simulink model "amplifierboard"  (R2020b)
settings: Solver=FixedStepDiscrete  StartTime=0.0  StopTime=2  FixedStep=0.01  RelTol=1e-3
InitFcn:
  | mbd_s32k_consistency_checks(bdroot(gcs));
undefined symbols (not defined in the file): AutoLowerVal, AutoRaiseVal, HoldVal, LED_En, LED_Off, LED_On, Logic_High, Logic_Low, LQFP, ManualLowerVal, ManualRaiseVal, PWRWNDW_CHDLCK, sC_bool_PWMEN, sC_cnt_FWSetting, sC_cnt_Mtr_DrvNo_HB, sC_cnt_PWMHB1to4, sC_cnt_PWMHB5to8, sC_cnt_TargetSlowRange, sC_pct_ManualMax, sC_pct_RampDwn, sC_pct_RampUp, sC_pct_StartPWM, sC_pct_Targetmax, SwitchPackRangeOffset, Threshold_Value, Tolerant_Time
libraries: mbd_s32k1xx_ec_toolbox x205, simulink x59, canmsglib x19, Filter x15, wndwcmd x3
(part 5 of 6)

== system amplifierboard/CAN_Pack_And_Send/RRWndwCntDetect/SwtchPosDetect/RR_Dwn_CntDetect ==
  In6 : Inport
  Data Store Read3 : DataStoreRead  DataStoreName=RR_WindSw_Dwn_Cnts_Low
  Data Store Read4 : DataStoreRead  DataStoreName=RR_WindSw_Dwn_Cnts_Hi
  Logical Operator6 : Logic  AllPortsSameDT=off  OutDataTypeStr=boolean
  Relational Operator11 : RelationalOperator  Operator=<=  OutDataTypeStr=boolean  RndMeth=Simplest
  Relational Operator13 : RelationalOperator  OutDataTypeStr=boolean  RndMeth=Simplest
  Out6 : Outport
  wires:
  Logical Operator6/1 -> Out6/1  "Out"
  Data Store Read4/1 -> Relational Operator11/2
  Data Store Read3/1 -> Relational Operator13/2
  Relational Operator13/1 -> Logical Operator6/2
  Relational Operator11/1 -> Logical Operator6/1
  In6/1 -> Relational Operator11/1, Relational Operator13/1  "In"

== system amplifierboard/CAN_Pack_And_Send/RRWndwCntDetect/SwtchPosDetect/RR_ExpDwn_CntDetect ==
  SwitchCount1 : Inport
  Data Store Read1 : DataStoreRead  DataStoreName=RR_WindSw_ExpDwn_Cnts_Low
  Data Store Read2 : DataStoreRead  DataStoreName=RR_WindSw_ExpDwn_Cnts_Hi
  Logical Operator5 : Logic  AllPortsSameDT=off  OutDataTypeStr=boolean
  Relational Operator10 : RelationalOperator  Operator=<=  OutDataTypeStr=boolean  RndMeth=Simplest
  Relational Operator12 : RelationalOperator  OutDataTypeStr=boolean  RndMeth=Simplest
  Out5 : Outport
  wires:
  Data Store Read1/1 -> Relational Operator12/2
  SwitchCount1/1 -> Relational Operator10/1, Relational Operator12/1  "In"
  Relational Operator10/1 -> Logical Operator5/1
  Data Store Read2/1 -> Relational Operator10/2
  Logical Operator5/1 -> Out5/1  "Out"
  Relational Operator12/1 -> Logical Operator5/2

== system amplifierboard/CAN_Pack_And_Send/RRWndwCntDetect/SwtchPosDetect/RR_ExpUp_CntDetect ==
  In7 : Inport
  Data Store Read5 : DataStoreRead  DataStoreName=RR_WindSw_ExpUp_Cnts_Low
  Data Store Read6 : DataStoreRead  DataStoreName=RR_WindSw_ExpUp_Cnts_Hi
  Logical Operator7 : Logic  AllPortsSameDT=off  OutDataTypeStr=boolean
  Relational Operator14 : RelationalOperator  Operator=<=  OutDataTypeStr=boolean  RndMeth=Simplest
  Relational Operator15 : RelationalOperator  OutDataTypeStr=boolean  RndMeth=Simplest
  AutoRaiseCnt : Outport
  wires:
  Data Store Read5/1 -> Relational Operator15/2
  Relational Operator15/1 -> Logical Operator7/2
  Data Store Read6/1 -> Relational Operator14/2
  In7/1 -> Relational Operator14/1, Relational Operator15/1  "In"
  Logical Operator7/1 -> AutoRaiseCnt/1  "Out"
  Relational Operator14/1 -> Logical Operator7/1

== system amplifierboard/CAN_Pack_And_Send/RRWndwCntDetect/SwtchPosDetect/RR_NrmOpen_CntDetect ==
  In9 : Inport
  Data Store Read10 : DataStoreRead  DataStoreName=RR_WindSw_NrmOpen_Cnts_Hi
  Data Store Read9 : DataStoreRead  DataStoreName=RR_WindSw_NrmOpen_Cnts_Low
  Logical Operator9 : Logic  AllPortsSameDT=off  OutDataTypeStr=boolean
  Relational Operator18 : RelationalOperator  Operator=<=  OutDataTypeStr=boolean  RndMeth=Simplest
  Relational Operator19 : RelationalOperator  OutDataTypeStr=boolean  RndMeth=Simplest
  HoldCnt : Outport
  wires:
  Relational Operator19/1 -> Logical Operator9/2
  Data Store Read9/1 -> Relational Operator19/2
  Relational Operator18/1 -> Logical Operator9/1
  Data Store Read10/1 -> Relational Operator18/2
  Logical Operator9/1 -> HoldCnt/1  "Out"
  In9/1 -> Relational Operator18/1, Relational Operator19/1  "In"

== system amplifierboard/CAN_Pack_And_Send/RRWndwCntDetect/SwtchPosDetect/RR_Up_CntDetect ==
  In8 : Inport
  Data Store Read7 : DataStoreRead  DataStoreName=RR_WindSw_Up_Cnts_Low
  Data Store Read8 : DataStoreRead  DataStoreName=RR_WindSw_Up_Cnts_Hi
  Logical Operator8 : Logic  AllPortsSameDT=off  OutDataTypeStr=boolean
  Relational Operator16 : RelationalOperator  Operator=<=  OutDataTypeStr=boolean  RndMeth=Simplest
  Relational Operator17 : RelationalOperator  OutDataTypeStr=boolean  RndMeth=Simplest
  Out8 : Outport
  wires:
  Relational Operator16/1 -> Logical Operator8/1
  Logical Operator8/1 -> Out8/1  "Out"
  Data Store Read8/1 -> Relational Operator16/2
  Data Store Read7/1 -> Relational Operator17/2
  In8/1 -> Relational Operator16/1, Relational Operator17/1  "In"
  Relational Operator17/1 -> Logical Operator8/2

== system amplifierboard/CAN_Pack_And_Send/RRWndwCntDetect/SwtchPosDetect/SwitchPosDetect1 ==
  ManRaiseCnt : Inport
  ManLowerCnt : Inport  Port=2
  AutoRaiseCnt : Inport  Port=3
  AutoLowerCnt : Inport  Port=4
  HoldCnt : Inport  Port=5
  SwitchCount : Inport  Port=6
  AutoLowerVal : Constant  Value=AutoLowerVal
  AutoRaiseVal : Constant  Value=AutoRaiseVal
  HoldVal : Constant  Value=HoldVal
  ManualLowerVal : Constant  Value=ManualLowerVal
  ManualRaiseVal : Constant  Value=ManualRaiseVal
  Switch{,1..4} (5 alike) : Switch  Criteria=u2 ~= 0
  AvgCount : Outport
  wires:
  SwitchCount/1 -> Switch4/3  "SwitchCount"
  Switch4/1 -> Switch3/3
  HoldCnt/1 -> Switch4/2  "HoldCnt"
  ManLowerCnt/1 -> Switch1/2  "ManLowerCnt"
  AutoLowerCnt/1 -> Switch3/2  "AutoLowerCnt"
  Switch/1 -> AvgCount/1  "AvgCount"
  ManRaiseCnt/1 -> Switch/2  "ManRaiseCnt"
  ManualRaiseVal/1 -> Switch/1
  HoldVal/1 -> Switch4/1
  ManualLowerVal/1 -> Switch1/1
  AutoLowerVal/1 -> Switch3/1
  AutoRaiseVal/1 -> Switch2/1
  Switch3/1 -> Switch2/3
  Switch2/1 -> Switch1/3
  Switch1/1 -> Switch/3
  AutoRaiseCnt/1 -> Switch2/2  "AutoRaiseCnt"

== system amplifierboard/CAN_Receive_And_Unpack/Subsystem/Chart/CalibrateSwitchPack.ReadSwitchAtUpPosition/Generate_Data ==
  Constant1 : Constant  Value=0x00  OutDataTypeStr=uint8
  Constant2 : Constant  Value=0x04  OutDataTypeStr=uint8
  Constant3 : Constant  Value=0x71  OutDataTypeStr=uint8
  Constant4 : Constant  Value=0x01  OutDataTypeStr=uint8
  Constant5 : Constant  Value=0xA1  OutDataTypeStr=uint8
  Constant6 : Constant  Value=0x04  OutDataTypeStr=uint8
  Constant7 : Constant  Value=0x55  OutDataTypeStr=uint8
  Constant8 : Constant  Value=0x55  OutDataTypeStr=uint8
  Mux : Mux  Inputs=8
  Width : Width  DataType=uint8
  Data : Outport
  Length : Outport  Port=2
  wires:
  Mux/1 -> Width/1, Data/1
  Constant2/1 -> Mux/1
  Constant3/1 -> Mux/2
  Constant5/1 -> Mux/4
  Constant1/1 -> Mux/5
  Constant4/1 -> Mux/3
  Constant6/1 -> Mux/6
  Constant7/1 -> Mux/7
  Constant8/1 -> Mux/8
  Width/1 -> Length/1

== system amplifierboard/CAN_Receive_And_Unpack/Subsystem/Chart/CalibrateSwitchPack.SendPos31Response/Generate_Data ==
  Constant1 : Constant  Value=0x02  OutDataTypeStr=uint8
  Constant2 : Constant  Value=0x04  OutDataTypeStr=uint8
  Constant3 : Constant  Value=0x71  OutDataTypeStr=uint8
  Constant4 : Constant  Value=0x01  OutDataTypeStr=uint8
  Constant5 : Constant  Value=0xA1  OutDataTypeStr=uint8
  Constant6 : Constant  Value=0x55  OutDataTypeStr=uint8
  Constant7 : Constant  Value=0x55  OutDataTypeStr=uint8
  Constant8 : Constant  Value=0x55  OutDataTypeStr=uint8
  Mux : Mux  Inputs=8
  Width : Width  DataType=uint8
  Data : Outport
  Length : Outport  Port=2
  wires:
  Mux/1 -> Width/1, Data/1
  Constant2/1 -> Mux/1
  Constant3/1 -> Mux/2
  Constant5/1 -> Mux/4
  Constant1/1 -> Mux/5
  Constant4/1 -> Mux/3
  Constant6/1 -> Mux/6
  Constant7/1 -> Mux/7
  Constant8/1 -> Mux/8
  Width/1 -> Length/1

== system amplifierboard/CAN_Receive_And_Unpack/Subsystem/Chart/CalibrateSwitchPack.SendPos31Response2/Generate_Data ==
  Constant1 : Constant  Value=0x02  OutDataTypeStr=uint8
  Constant2 : Constant  Value=0x04  OutDataTypeStr=uint8
  Constant3 : Constant  Value=0x71  OutDataTypeStr=uint8
  Constant4 : Constant  Value=0x01  OutDataTypeStr=uint8
  Constant5 : Constant  Value=0xA1  OutDataTypeStr=uint8
  Constant6 : Constant  Value=0x55  OutDataTypeStr=uint8
  Constant7 : Constant  Value=0x55  OutDataTypeStr=uint8
  Constant8 : Constant  Value=0x55  OutDataTypeStr=uint8
  Mux : Mux  Inputs=8
  Width : Width  DataType=uint8
  Data : Outport
  Length : Outport  Port=2
  wires:
  Mux/1 -> Width/1, Data/1
  Constant2/1 -> Mux/1
  Constant3/1 -> Mux/2
  Constant5/1 -> Mux/4
  Constant1/1 -> Mux/5
  Constant4/1 -> Mux/3
  Constant6/1 -> Mux/6
  Constant7/1 -> Mux/7
  Constant8/1 -> Mux/8
  Width/1 -> Length/1

== system amplifierboard/CAN_Receive_And_Unpack/Subsystem/Chart/CalibrateSwitchPack.SendPos31StopPosResp/Generate_Data ==
  Constant1 : Constant  Value=0x02  OutDataTypeStr=uint8
  Constant2 : Constant  Value=0x04  OutDataTypeStr=uint8
  Constant3 : Constant  Value=0x71  OutDataTypeStr=uint8
  Constant4 : Constant  Value=0x02  OutDataTypeStr=uint8
  Constant5 : Constant  Value=0xA1  OutDataTypeStr=uint8
  Constant6 : Constant  Value=0x55  OutDataTypeStr=uint8
  Constant7 : Constant  Value=0x55  OutDataTypeStr=uint8
  Constant8 : Constant  Value=0x55  OutDataTypeStr=uint8
  Mux : Mux  Inputs=8
  Width : Width  DataType=uint8
  Data : Outport
  Length : Outport  Port=2
  wires:
  Mux/1 -> Width/1, Data/1
  Constant2/1 -> Mux/1
  Constant3/1 -> Mux/2
  Constant5/1 -> Mux/4
  Constant1/1 -> Mux/5
  Constant4/1 -> Mux/3
  Constant6/1 -> Mux/6
  Constant7/1 -> Mux/7
  Constant8/1 -> Mux/8
  Width/1 -> Length/1

== system amplifierboard/CAN_Receive_And_Unpack/Subsystem/Chart/SendNeg2EResponse/Generate_Data ==
  Constant{1,6..8} (4 alike) : Constant  Value=0x55  OutDataTypeStr=uint8
  Constant2 : Constant  Value=0x03  OutDataTypeStr=uint8
  Constant3 : Constant  Value=0x7F  OutDataTypeStr=uint8
  Constant4 : Constant  Value=0x2E  OutDataTypeStr=uint8
  Constant5 : Constant  Value=0x12  OutDataTypeStr=uint8
  Mux : Mux  Inputs=8
  Width : Width  DataType=uint8
  Data : Outport
  Length : Outport  Port=2
  wires:
  Mux/1 -> Width/1, Data/1
  Constant2/1 -> Mux/1
  Constant3/1 -> Mux/2
  Constant5/1 -> Mux/4
  Constant1/1 -> Mux/5
  Constant4/1 -> Mux/3
  Constant6/1 -> Mux/6
  Constant7/1 -> Mux/7
  Constant8/1 -> Mux/8
  Width/1 -> Length/1

== system amplifierboard/CAN_Receive_And_Unpack/Subsystem/Chart/SendPos11Resp/Generate_Data ==
  Constant{1,5..8} (5 alike) : Constant  Value=0x55  OutDataTypeStr=uint8
  Constant2 : Constant  Value=0x02  OutDataTypeStr=uint8
  Constant3 : Constant  Value=0x51  OutDataTypeStr=uint8
  Constant4 : Constant  Value=0x02  OutDataTypeStr=uint8
  Mux : Mux  Inputs=8
  Width : Width  DataType=uint8
  Data : Outport
  Length : Outport  Port=2
  wires:
  Mux/1 -> Width/1, Data/1
  Constant2/1 -> Mux/1
  Constant3/1 -> Mux/2
  Constant5/1 -> Mux/4
  Constant1/1 -> Mux/5
  Constant4/1 -> Mux/3
  Constant6/1 -> Mux/6
  Constant7/1 -> Mux/7
  Constant8/1 -> Mux/8
  Width/1 -> Length/1

== system amplifierboard/CAN_Receive_And_Unpack/Subsystem/Chart/SendPos22Resp_SW_Ver/Generate_Data ==
  Constant2 : Constant  Value=0x0B  OutDataTypeStr=uint8
  Constant3 : Constant  Value=0x62  OutDataTypeStr=uint8
  Constant4 : Constant  Value=0x01  OutDataTypeStr=uint8
  Constant5 : Constant  Value=0x00  OutDataTypeStr=uint8
  DataMemRead : mbd_s32k1xx_ec_toolbox/Utility Blocks/DataMemRead  base=0x1FFFFFF0  offset=0x0000  ptr=uint8_t
  DataMemRead1 : mbd_s32k1xx_ec_toolbox/Utility Blocks/DataMemRead  base=0x1FFFFFF0  offset=0x0001  ptr=uint8_t
  DataMemRead2 : mbd_s32k1xx_ec_toolbox/Utility Blocks/DataMemRead  base=0x1FFFFFF0  offset=0x0002  ptr=uint8_t
  DataMemRead3 : mbd_s32k1xx_ec_toolbox/Utility Blocks/DataMemRead  base=0x1FFFFFF0  offset=0x0003  ptr=uint8_t
  Mux : Mux  Inputs=8
  Width : Width  DataType=uint8
  Data : Outport
  Length : Outport  Port=2
  wires:
  Mux/1 -> Width/1, Data/1
  Constant2/1 -> Mux/1
  Constant3/1 -> Mux/2
  Constant5/1 -> Mux/4
  DataMemRead/1 -> Mux/5
  Constant4/1 -> Mux/3
  DataMemRead1/1 -> Mux/6
  DataMemRead2/1 -> Mux/7
  DataMemRead3/1 -> Mux/8
  Width/1 -> Length/1

== system amplifierboard/CAN_Receive_And_Unpack/Subsystem/Chart/SendPos22Resp_SW_Ver1/Generate_Data ==
  Constant1 : Constant  Value=0x55  OutDataTypeStr=uint8
  Constant2 : Constant  Value=0x30  OutDataTypeStr=uint8
  Constant3 : Constant  Value=0x55  OutDataTypeStr=uint8
  Constant5 : Constant  Value=0x55  OutDataTypeStr=uint8
  DataMemRead4 : mbd_s32k1xx_ec_toolbox/Utility Blocks/DataMemRead  base=0x1FFFFFF0  offset=0x0004  ptr=uint8_t
  DataMemRead5 : mbd_s32k1xx_ec_toolbox/Utility Blocks/DataMemRead  base=0x1FFFFFF0  offset=0x0005  ptr=uint8_t
  DataMemRead6 : mbd_s32k1xx_ec_toolbox/Utility Blocks/DataMemRead  base=0x1FFFFFF0  offset=0x0006  ptr=uint8_t
  DataMemRead7 : mbd_s32k1xx_ec_toolbox/Utility Blocks/DataMemRead  base=0x1FFFFFF0  offset=0x0007  ptr=uint8_t
  Mux : Mux  Inputs=8
  Width : Width  DataType=uint8
  Data : Outport
  Length : Outport  Port=2
  wires:
  Mux/1 -> Width/1, Data/1
  Constant2/1 -> Mux/1
  Width/1 -> Length/1
  DataMemRead4/1 -> Mux/2
  DataMemRead6/1 -> Mux/4
  DataMemRead7/1 -> Mux/5
  DataMemRead5/1 -> Mux/3
  Constant5/1 -> Mux/8
  Constant3/1 -> Mux/7
  Constant1/1 -> Mux/6

== system amplifierboard/CAN_Receive_And_Unpack/Subsystem/Chart/SendPos2EResponse/Generate_Data ==
  Constant{1,6..8} (4 alike) : Constant  Value=0x55  OutDataTypeStr=uint8
  Constant2 : Constant  Value=0x03  OutDataTypeStr=uint8
  Constant3 : Constant  Value=0x6E  OutDataTypeStr=uint8
  Constant4 : Constant  Value=0x01  OutDataTypeStr=uint8
  Constant5 : Constant  Value=0x01  OutDataTypeStr=uint8
  Mux : Mux  Inputs=8
  Width : Width  DataType=uint8
  Data : Outport
  Length : Outport  Port=2
  wires:
  Mux/1 -> Width/1, Data/1
  Constant2/1 -> Mux/1
  Constant3/1 -> Mux/2
  Constant5/1 -> Mux/4
  Constant1/1 -> Mux/5
  Constant4/1 -> Mux/3
  Constant6/1 -> Mux/6
  Constant7/1 -> Mux/7
  Constant8/1 -> Mux/8
  Width/1 -> Length/1

== system amplifierboard/CAN_Receive_And_Unpack/Subsystem/Chart/SendPos31StopPosResp/Generate_Data ==
  Constant1 : Constant  Value=0x02  OutDataTypeStr=uint8
  Constant2 : Constant  Value=0x04  OutDataTypeStr=uint8
  Constant3 : Constant  Value=0x71  OutDataTypeStr=uint8
  Constant4 : Constant  Value=0x02  OutDataTypeStr=uint8
  Constant5 : Constant  Value=0xA1  OutDataTypeStr=uint8
  Constant6 : Constant  Value=0x55  OutDataTypeStr=uint8
  Constant7 : Constant  Value=0x55  OutDataTypeStr=uint8
  Constant8 : Constant  Value=0x55  OutDataTypeStr=uint8
  Mux : Mux  Inputs=8
  Width : Width  DataType=uint8
  Data : Outport
  Length : Outport  Port=2
  wires:
  Mux/1 -> Width/1, Data/1
  Constant2/1 -> Mux/1
  Constant3/1 -> Mux/2
  Constant5/1 -> Mux/4
  Constant1/1 -> Mux/5
  Constant4/1 -> Mux/3
  Constant6/1 -> Mux/6
  Constant7/1 -> Mux/7
  Constant8/1 -> Mux/8
  Width/1 -> Length/1

== system amplifierboard/CAN_Receive_And_Unpack/Subsystem1/Fold_Unfold/If Action Subsystem ==
  Action Port : ActionPort  ActionPortLabel=if(u1 == 1)
  Forward : Constant  OutDataTypeStr=int8
  "Forward_Direction " : Outport
  wires:
  Forward/1 -> "Forward_Direction "/1

== system amplifierboard/CAN_Receive_And_Unpack/Subsystem1/Fold_Unfold/If Action Subsystem1 ==
  Action Port : ActionPort  ActionPortLabel=elseif(u2 == 1)
  Reverse : Constant  Value=-1  OutDataTypeStr=int8
  Reverse_Direction : Outport
  wires:
  Reverse/1 -> Reverse_Direction/1

== system amplifierboard/CAN_Receive_And_Unpack/Subsystem1/Fold_Unfold/If Action Subsystem2 ==
  Action Port : ActionPort  ActionPortLabel=elseif( u3 == 1 )
  Standstill : Constant  Value=0  OutDataTypeStr=int8
  Standstill_Invalid : Outport
  wires:
  Standstill/1 -> Standstill_Invalid/1

== system amplifierboard/CAN_Receive_And_Unpack/Subsystem1/Fold_Unfold/If Action Subsystem3 ==
  Action Port : ActionPort  ActionPortLabel=elseif( u4 == 1 )
  Standstill : Constant  Value=0  OutDataTypeStr=int8
  Standstill_invalid : Outport
  wires:
  Standstill/1 -> Standstill_invalid/1

== system amplifierboard/CAN_Receive_And_Unpack/Subsystem1/Motor4/If Action Subsystem ==
  Action Port : ActionPort  ActionPortLabel=if(u1 == 1)
  Forward : Constant  OutDataTypeStr=int8
  "Forward_Direction " : Outport
  wires:
  Forward/1 -> "Forward_Direction "/1

== system amplifierboard/CAN_Receive_And_Unpack/Subsystem1/Motor4/If Action Subsystem1 ==
  Action Port : ActionPort  ActionPortLabel=elseif(u2 == 1)
  Reverse : Constant  Value=-1  OutDataTypeStr=int8
  Reverse_Direction : Outport
  wires:
  Reverse/1 -> Reverse_Direction/1

== system amplifierboard/CAN_Receive_And_Unpack/Subsystem1/Motor4/If Action Subsystem2 ==
  Action Port : ActionPort  ActionPortLabel=elseif( u3 == 1 )
  Standstill : Constant  Value=0  OutDataTypeStr=int8
  Standstill_Invalid : Outport
  wires:
  Standstill/1 -> Standstill_Invalid/1

== system amplifierboard/CAN_Receive_And_Unpack/Subsystem1/Motor4/If Action Subsystem3 ==
  Action Port : ActionPort  ActionPortLabel=elseif( u4 == 1 )
  Standstill : Constant  Value=0  OutDataTypeStr=int8
  Standstill_invalid : Outport
  wires:
  Standstill/1 -> Standstill_invalid/1

== system amplifierboard/CAN_Receive_And_Unpack/Subsystem1/Motor5/If Action Subsystem ==
  Action Port : ActionPort  ActionPortLabel=if(u2 == 1)
  Forward : Constant  Value=-1  OutDataTypeStr=int8
  "Forward_Direction " : Outport
  wires:
  Forward/1 -> "Forward_Direction "/1

== system amplifierboard/CAN_Receive_And_Unpack/Subsystem1/Motor5/If Action Subsystem1 ==
  Action Port : ActionPort  ActionPortLabel=else
  Standstill : Constant  Value=0  OutDataTypeStr=int8
  Standstill_Invalid : Outport
  wires:
  Standstill/1 -> Standstill_Invalid/1

== system amplifierboard/CAN_Receive_And_Unpack/Subsystem1/Motor6/If Action Subsystem ==
  Action Port : ActionPort  ActionPortLabel=if(u1 == 1)
  Forward : Constant  OutDataTypeStr=int8
  "Forward_Direction " : Outport
  wires:
  Forward/1 -> "Forward_Direction "/1

== system amplifierboard/CAN_Receive_And_Unpack/Subsystem1/Motor6/If Action Subsystem1 ==
  Action Port : ActionPort  ActionPortLabel=elseif(u2 == 1)
  Reverse : Constant  Value=-1  OutDataTypeStr=int8
  Reverse_Direction : Outport
  wires:
  Reverse/1 -> Reverse_Direction/1

== system amplifierboard/CAN_Receive_And_Unpack/Subsystem1/Motor6/If Action Subsystem2 ==
  Action Port : ActionPort  ActionPortLabel=elseif( u3 == 1 )
  Standstill : Constant  Value=0  OutDataTypeStr=int8
  Standstill_Invalid : Outport
  wires:
  Standstill/1 -> Standstill_Invalid/1

== system amplifierboard/CAN_Receive_And_Unpack/Subsystem1/Motor6/If Action Subsystem3 ==
  Action Port : ActionPort  ActionPortLabel=elseif( u4 == 1 )
  Standstill : Constant  Value=0  OutDataTypeStr=int8
  Standstill_invalid : Outport
  wires:
  Standstill/1 -> Standstill_invalid/1

== system amplifierboard/CAN_Receive_And_Unpack/Subsystem1/Subsystem1/Motor2 ==
  Input : Inport
  Input1 : Inport  Port=2
  Compare To Constant : simulink/Logic and Bit Operations/Compare To Constant  relop===  const=1.0  OutDataTypeStr=boolean
  Compare To Constant{1..2,4..5} (4 alike) : simulink/Logic and Bit Operations/Compare To Constant  relop===  const=0  OutDataTypeStr=boolean
  Compare To Constant3 : simulink/Logic and Bit Operations/Compare To Constant  relop===  const=1  OutDataTypeStr=boolean
  Compare To Constant6 : simulink/Logic and Bit Operations/Compare To Constant  relop===  const=1  OutDataTypeStr=boolean
  Compare To Constant7 : simulink/Logic and Bit Operations/Compare To Constant  relop===  const=1  OutDataTypeStr=boolean
  If : If  NumInputs=4  IfExpression=u1 == 1  ElseIfExpressions=u2 == 1, u3 == 1 , u4 == 1  ShowElse=off
  If Action Subsystem : Subsystem  TreatAsAtomicUnit=on
  If Action Subsystem1 : Subsystem  TreatAsAtomicUnit=on
  If Action Subsystem2 : Subsystem  TreatAsAtomicUnit=on
  If Action Subsystem3 : Subsystem  TreatAsAtomicUnit=on
  Logical Operator{,1..3} (4 alike) : Logic  AllPortsSameDT=off  OutDataTypeStr=boolean
  Merge : Merge  Inputs=4
  Motor : Outport
  wires:
  Logical Operator/1 -> If/1
  If/3 -> If Action Subsystem2/Action
  Compare To Constant1/1 -> Logical Operator/2
  Logical Operator1/1 -> If/2
  Logical Operator2/1 -> If/3
  If/1 -> If Action Subsystem/Action
  If Action Subsystem2/1(Standstill_Invalid) -> Merge/3
  If Action Subsystem3/1(Standstill_invalid) -> Merge/4
  If Action Subsystem1/1(Reverse_Direction) -> Merge/2
  Merge/1 -> Motor/1
  Compare To Constant6/1 -> Logical Operator3/1
  If/4 -> If Action Subsystem3/Action
  Compare To Constant7/1 -> Logical Operator3/2
  Input/1 -> Compare To Constant/1, Compare To Constant6/1, Compare To Constant4/1, Compare To Constant2/1
  Logical Operator3/1 -> If/4
  Compare To Constant/1 -> Logical Operator/1
  Compare To Constant3/1 -> Logical Operator1/2
  Compare To Constant4/1 -> Logical Operator2/1
  Compare To Constant2/1 -> Logical Operator1/1
  If/2 -> If Action Subsystem1/Action
  If Action Subsystem/1("Forward_Direction ") -> Merge/1
  Compare To Constant5/1 -> Logical Operator2/2
  Input1/1 -> Compare To Constant1/1, Compare To Constant3/1, Compare To Constant5/1, Compare To Constant7/1

== system amplifierboard/CAN_Receive_And_Unpack/Subsystem1/Subsystem1/Motor3 ==
  Input : Inport
  Input1 : Inport  Port=2
  Compare To Constant : simulink/Logic and Bit Operations/Compare To Constant  relop===  const=1.0  OutDataTypeStr=boolean
  Compare To Constant{1..2,4..5} (4 alike) : simulink/Logic and Bit Operations/Compare To Constant  relop===  const=0  OutDataTypeStr=boolean
  Compare To Constant3 : simulink/Logic and Bit Operations/Compare To Constant  relop===  const=1  OutDataTypeStr=boolean
  Compare To Constant6 : simulink/Logic and Bit Operations/Compare To Constant  relop===  const=1  OutDataTypeStr=boolean
  Compare To Constant7 : simulink/Logic and Bit Operations/Compare To Constant  relop===  const=1  OutDataTypeStr=boolean
  If : If  NumInputs=4  IfExpression=u1 == 1  ElseIfExpressions=u2 == 1, u3 == 1 , u4 == 1  ShowElse=off
  If Action Subsystem : Subsystem  TreatAsAtomicUnit=on
  If Action Subsystem1 : Subsystem  TreatAsAtomicUnit=on
  If Action Subsystem2 : Subsystem  TreatAsAtomicUnit=on
  If Action Subsystem3 : Subsystem  TreatAsAtomicUnit=on
  Logical Operator{,1..3} (4 alike) : Logic  AllPortsSameDT=off  OutDataTypeStr=boolean
  Merge : Merge  Inputs=4
  Motor : Outport
  wires:
  Input1/1 -> Compare To Constant7/1, Compare To Constant5/1, Compare To Constant3/1, Compare To Constant1/1
  Compare To Constant5/1 -> Logical Operator2/2
  If Action Subsystem/1("Forward_Direction ") -> Merge/1
  If/2 -> If Action Subsystem1/Action
  Compare To Constant2/1 -> Logical Operator1/1
  Compare To Constant4/1 -> Logical Operator2/1
  Compare To Constant3/1 -> Logical Operator1/2
  Compare To Constant/1 -> Logical Operator/1
  Logical Operator3/1 -> If/4
  Input/1 -> Compare To Constant2/1, Compare To Constant4/1, Compare To Constant6/1, Compare To Constant/1
  Compare To Constant7/1 -> Logical Operator3/2
  If/4 -> If Action Subsystem3/Action
  Compare To Constant6/1 -> Logical Operator3/1
  Merge/1 -> Motor/1
  If Action Subsystem1/1(Reverse_Direction) -> Merge/2
  If Action Subsystem3/1(Standstill_invalid) -> Merge/4
  If Action Subsystem2/1(Standstill_Invalid) -> Merge/3
  If/1 -> If Action Subsystem/Action
  Logical Operator2/1 -> If/3
  Logical Operator1/1 -> If/2
  Compare To Constant1/1 -> Logical Operator/2
  If/3 -> If Action Subsystem2/Action
  Logical Operator/1 -> If/1

== system amplifierboard/Motor_Control/Motor_Control/Chart/SendSPI/Switch Case Action Subsystem ==
  SPI_Command1 : Inport  OutDataTypeStr=uint8  PortDimensions=[1 2]
  Action Port : ActionPort  ActionPortLabel=case [ 1 ]:
  LPSPI_Master_Transfer : mbd_s32k1xx_ec_toolbox/Communication Blocks/SPI Blocks/LPSPI_Master_Transfer  instance=2  pcs=0  pcs_polarity=ActiveLow  xfermode=Blocking  timeout=50  spi_upd=on
  Status_Out1 : Outport  OutDataTypeStr=uint8
  wires:
  SPI_Command1/1 -> LPSPI_Master_Transfer/1
  LPSPI_Master_Transfer/1 -> Status_Out1/1

== system amplifierboard/Motor_Control/Motor_Control/Chart/SendSPI/Switch Case Action Subsystem1 ==
  SPI_Command2 : Inport  OutDataTypeStr=uint8  PortDimensions=[1 2]
  Action Port : ActionPort  ActionPortLabel=case [ 2 ]:
  LPSPI_Master_Transfer : mbd_s32k1xx_ec_toolbox/Communication Blocks/SPI Blocks/LPSPI_Master_Transfer  instance=1  pcs=1  pcs_polarity=ActiveLow  xfermode=Blocking  timeout=50  spi_upd=on
  Status_Out2 : Outport  OutDataTypeStr=uint8
  wires:
  LPSPI_Master_Transfer/1 -> Status_Out2/1
  SPI_Command2/1 -> LPSPI_Master_Transfer/1

== system amplifierboard/CAN_Receive_And_Unpack/Subsystem1/Subsystem1/Motor2/If Action Subsystem ==
  Action Port : ActionPort  ActionPortLabel=if(u1 == 1)
  Forward : Constant  OutDataTypeStr=int8
  "Forward_Direction " : Outport
  wires:
  Forward/1 -> "Forward_Direction "/1

== system amplifierboard/CAN_Receive_And_Unpack/Subsystem1/Subsystem1/Motor2/If Action Subsystem1 ==
  Action Port : ActionPort  ActionPortLabel=elseif(u2 == 1)
  Reverse : Constant  Value=-1  OutDataTypeStr=int8
  Reverse_Direction : Outport
  wires:
  Reverse/1 -> Reverse_Direction/1

== system amplifierboard/CAN_Receive_And_Unpack/Subsystem1/Subsystem1/Motor2/If Action Subsystem2 ==
  Action Port : ActionPort  ActionPortLabel=elseif( u3 == 1 )
  Standstill : Constant  Value=0  OutDataTypeStr=int8
  Standstill_Invalid : Outport
  wires:
  Standstill/1 -> Standstill_Invalid/1

== system amplifierboard/CAN_Receive_And_Unpack/Subsystem1/Subsystem1/Motor2/If Action Subsystem3 ==
  Action Port : ActionPort  ActionPortLabel=elseif( u4 == 1 )
  Standstill : Constant  Value=0  OutDataTypeStr=int8
  Standstill_invalid : Outport
  wires:
  Standstill/1 -> Standstill_invalid/1

== system amplifierboard/CAN_Receive_And_Unpack/Subsystem1/Subsystem1/Motor3/If Action Subsystem ==
  Action Port : ActionPort  ActionPortLabel=if(u1 == 1)
  Forward : Constant  OutDataTypeStr=int8
  "Forward_Direction " : Outport
  wires:
  Forward/1 -> "Forward_Direction "/1

== system amplifierboard/CAN_Receive_And_Unpack/Subsystem1/Subsystem1/Motor3/If Action Subsystem1 ==
  Action Port : ActionPort  ActionPortLabel=elseif(u2 == 1)
  Reverse : Constant  Value=-1  OutDataTypeStr=int8
  Reverse_Direction : Outport
  wires:
  Reverse/1 -> Reverse_Direction/1

== system amplifierboard/CAN_Receive_And_Unpack/Subsystem1/Subsystem1/Motor3/If Action Subsystem2 ==
  Action Port : ActionPort  ActionPortLabel=elseif( u3 == 1 )
  Standstill : Constant  Value=0  OutDataTypeStr=int8
  Standstill_Invalid : Outport
  wires:
  Standstill/1 -> Standstill_Invalid/1

== system amplifierboard/CAN_Receive_And_Unpack/Subsystem1/Subsystem1/Motor3/If Action Subsystem3 ==
  Action Port : ActionPort  ActionPortLabel=elseif( u4 == 1 )
  Standstill : Constant  Value=0  OutDataTypeStr=int8
  Standstill_invalid : Outport
  wires:
  Standstill/1 -> Standstill_invalid/1

== stateflow chart amplifierboard/CAN_Pack_And_Send/Trigger ==
  (default) -> (junction 125)
  (junction 125) -> (junction 127) [order 1] : [TX_Cnt < 5]
      | {TX_Cnt = TX_Cnt + 1;
      | bool_TX = false;}
      | %stop transmit
  (junction 127) -> (junction 92)
  (junction 125) -> (junction 92) [order 2] : {%set up to transmit message
      | bool_TX = true;
      | TX_Cnt = 0;}
  data: TX_Cnt local =0; bool_TX output

== stateflow chart amplifierboard/HALL_Input_Capture/Hall_Count_Calculation ==
  settings: executeAtInitialization=1
  (default) -> (junction 1100) : {Motor_idx = 0;}
  (junction 1100) -> (junction 1104) [order 1] : HE1
      | {Motor_idx = 1;}
  (junction 1100) -> (junction 1102) [order 2]
  (junction 1104) -> (junction 1106)
  (junction 1102) -> (junction 1106) [order 1] : HE2
      | {Motor_idx = 2;}
  (junction 1102) -> (junction 1112) [order 2]
  (junction 1106) -> (junction 1117)
  (junction 1112) -> (junction 1117) [order 1] : HE3
      | {Motor_idx = 3;}
  (junction 1112) -> (junction 1115) [order 2]
  (junction 1117) -> (junction 1111)
  (junction 1115) -> (junction 1111) [order 1] : HE4
      | {Motor_idx = 4;}
  (junction 1115) -> (junction 1126) [order 2]
  (junction 1111) -> (junction 1124)
  (junction 1126) -> (junction 1124) [order 1] : HE5
      | {Motor_idx = 5;}
  (junction 1126) -> (junction 1121) [order 2]
  (junction 1124) -> (junction 1123)
  (junction 1121) -> (junction 1123) [order 1] : HE6
      | {Motor_idx = 6;}
  (junction 1121) -> (junction 1157) [order 2]
  (junction 1123) -> (junction 1155)
  (junction 1157) -> (junction 1155) [order 1] : HE7
      | {Motor_idx = 7;}
  (junction 1157) -> (junction 1158) [order 2]
  (junction 1155) -> (junction 1156)
  (junction 1158) -> (junction 1156) [order 1] : HE8
      | {Motor_idx = 8;}
  (junction 1158) -> (junction 1147) [order 2] : Tick
  (junction 1156) -> (junction 1138) [order 2]
  (junction 1156) -> (junction 1138) [order 1] : [MotorPosCount(Motor_idx) > 1000]
      | {MotorPosRawCount(Motor_idx) = min(MotorPosRawCount(Motor_idx)+1,MotorPosMaxCount(Motor_idx));}
  (junction 1138) -> (junction 1147) [order 1] : [MotorPosCount(Motor_idx) < 0]
      | {MotorPosRawCount(Motor_idx) = max(MotorPosRawCount(Motor_idx)-1, 0);}
  (junction 1138) -> (junction 1147) [order 2]
  (junction 1147) -> (junction 1152) : {MotorPosCount= uint8((single(MotorPosRawCount)./single(MotorPosMaxCount))*254);}
  data: MotorPosCount output uint8 size=8 =zeros(8,1,'uint8'); Motor_idx local size=1 =0; MotorPosRawCount local uint16 size=8 =uint16([100;100;100;100;100;100;100;100]); MotorPosMaxCount local uint16 size=8 =uint16([1000;1000;1000;1000;1000;1000;1000;1000])
  events: HE1 input FUNCTION_CALL_EVENT; HE2 input FUNCTION_CALL_EVENT; HE3 input FUNCTION_CALL_EVENT; HE4 input FUNCTION_CALL_EVENT; HE5 input FUNCTION_CALL_EVENT; HE6 input FUNCTION_CALL_EVENT; HE7 input FUNCTION_CALL_EVENT; Tick input FUNCTION_CALL_EVENT; Trig_HallTrack input FUNCTION_CALL_EVENT; HE8 input FUNCTION_CALL_EVENT

== stateflow chart amplifierboard/Motor_Control/Subsystem/Chart ==
  state Idle
    PWM_Out = zeros(6,1,'single');
  state Assign
    en: PWM_Out = zeros(6,1,'single');
    Assign -> (junction 9) [order 1] : {for_idx = 1;}
    (junction 9) -> (junction 11) [order 1] : [for_idx < 7]
    (junction 11) -> (junction 18) [order 2]
    (junction 18) -> (junction 25) [order 2]
    (junction 25) -> (junction 30) [order 2]
    (junction 15) -> (junction 9) : {for_idx = for_idx + 1;}
    (junction 11) -> (junction 15) [order 1] : [aV_int_MotorDir(for_idx) == 0]
        | { PWM_Out(for_idx) = 0;}
    (junction 18) -> (junction 20) [order 1] : [aV_int_MotorDir(for_idx) == 1]
        | {PWM_Out(for_idx) = min(max((PWM_Out(for_idx)+RampUp),StartPWM),ManualMaxPWM);}
    (junction 25) -> (junction 27) [order 1] : [PositionError(for_idx) < TargetSlowRange]
        | {PWM_Out(for_idx) = max((PWM_Out(for_idx)-RampDwn), StartPWM);}
    (junction 30) -> (junction 32) : {PWM_Out(for_idx) = min(max((PWM_Out(for_idx)+RampUp),StartPWM),TargetMaxPWM);}
    (junction 9) -> (junction 13) [order 2]
    (junction 20) -> (junction 15)
    (junction 27) -> (junction 20)
    (junction 32) -> (junction 27)
  (default) -> Idle
  Idle -> Assign : [any(aV_int_MotorDir ~= 0)]
  Assign -> Idle [order 1] : [all(aV_int_MotorDir == 0)...
      | && all(PWM_Out == 0)]
  data: aV_int_MotorDir input int8 size=6; PositionError input uint8 size=6; PWM_Out output single size=6 =zeros(6,1,'single'); for_idx local size=1 =0; RampUp input single size=1; RampDwn input single size=1; StartPWM input single size=1; ManualMaxPWM input single size=1; TargetMaxPWM input single size=1; TargetSlowRange input uint16 size=1

== stateflow chart amplifierboard/CAN_Receive_And_Unpack/Subsystem/Chart ==
  settings: sampleTime=1
  state Idle
    StateFlowState=0;
  note: ?
  state ParseMessage
    StateFlowState=1;
    ContinueStateProcessing = 1;
  state Diagnostic_ID_req_Verified
    StateFlowState=1;
  state CalibrateSwitchPack
    state AcknowledgeSer31Request
      ContinueStateProcessing = 1;
      StateFlowState= 11;
    state WaitforCommand
      StateFlowState=12;
    state SendPos31Response1
    state SampleNO_SwitchState
      ReadSwitchAtNormOpen
      StateFlowState=13;
    state SendPos31Response [function]
    state CapturingDownSwitchValues
      ReadSwitchAtDownPostion
      StateFlowState=14;
    state ReadSwitchAtNormOpen [function]
    state ReadSwitchAtDownPostion [function]
    state CapturingExpDownSwitchValues
      ReadSwitchAtExpDownPosition
      StateFlowState=15;
    state ReadSwitchAtExpDownPosition [function]
    state CapturingUpSwitchValues
      ReadSwitchAtUpPosition
      StateFlowState=16;
    state ReadSwitchAtUpPosition [function]
    state ReadSwitchAtExpUpPosition [function]
    state SampleExpUp_SwitchState
      ReadSwitchAtExpUpPosition
      StateFlowState=17;
    state SendPos31StopPosResp [function]
    state ExitSer31CalSwPack
      WriteCalValuesToEEPROM
      StateFlowState=18;
    state SendPos31Response2 [function]
    state WriteCalValuesToEEPROM [function]
    state Exit
      StateFlowState=19;
      ContinueStateProcessing = 0;
    (default) -> AcknowledgeSer31Request
    AcknowledgeSer31Request -> WaitforCommand : after(10, msec){SendPos31Response}
    WaitforCommand -> SendPos31Response1 : [ (ServiceID == 0x31) && (ServiceByte0==0x01) && (ServiceByte1==0xA1) && (ServiceByte2==0x02)&& (ServiceByte3 ==0x01) ]{SendPos31Response}
    SendPos31Response1 -> SampleNO_SwitchState : after(10, msec)
    SampleNO_SwitchState -> CapturingDownSwitchValues [order 1] : [ (ServiceID == 0x31) && (ServiceByte0==0x01) && (ServiceByte1==0xA1) && (ServiceByte2==0x02)&& (ServiceByte3 ==0x02) ]{SendPos31Response}
    SampleNO_SwitchState -> ExitSer31CalSwPack [order 2] : [ (ServiceID == 0x31) && (ServiceByte0==0x02) && (ServiceByte1==0xA1) && (ServiceByte2==0x02) ]{SendPos31StopPosResp}
    CapturingDownSwitchValues -> ExitSer31CalSwPack [order 2] : [ (ServiceID == 0x31) && (ServiceByte0==0x02) && (ServiceByte1==0xA1) && (ServiceByte2==0x02) ]{SendPos31StopPosResp}
    CapturingDownSwitchValues -> CapturingExpDownSwitchValues [order 1] : [ (ServiceID == 0x31) && (ServiceByte0==0x01) && (ServiceByte1==0xA1) && (ServiceByte2==0x02)&& (ServiceByte3 ==0x03) ]{SendPos31Response}
    CapturingExpDownSwitchValues -> ExitSer31CalSwPack [order 2] : [ (ServiceID == 0x31) && (ServiceByte0==0x02) && (ServiceByte1==0xA1) && (ServiceByte2==0x02) ]{SendPos31StopPosResp}
    CapturingExpDownSwitchValues -> CapturingUpSwitchValues [order 1] : [ (ServiceID == 0x31) && (ServiceByte0==0x01) && (ServiceByte1==0xA1) && (ServiceByte2==0x02)&& (ServiceByte3 ==0x04) ]{SendPos31Response}
    CapturingUpSwitchValues -> ExitSer31CalSwPack [order 2] : [ (ServiceID == 0x31) && (ServiceByte0==0x02) && (ServiceByte1==0xA1) && (ServiceByte2==0x02) ]{SendPos31StopPosResp}
    CapturingUpSwitchValues -> SampleExpUp_SwitchState [order 1] : [ (ServiceID == 0x31) && (ServiceByte0==0x01) && (ServiceByte1==0xA1) && (ServiceByte2==0x02)&& (ServiceByte3 ==0x05) ]{SendPos31Response2}
    SampleExpUp_SwitchState -> ExitSer31CalSwPack : [ (ServiceID == 0x31) && (ServiceByte0==0x02) && (ServiceByte1==0xA1) && (ServiceByte2==0x02) ]{SendPos31StopPosResp}
    ExitSer31CalSwPack -> Exit : [ (ServiceID == 0x31) && (ServiceByte0==0x03) && (ServiceByte1==0xA1) && (ServiceByte2==0x02) ]
    Exit -> (junction 190)
  state SendNeg2EResponse [function]
  state SW_VersionRequest
    ContinueStateProcessing = 1;
    StateFlowState=9;
  state PositiveRespone
    StateFlowState=2;
  state SendPos2EResponse [function]
  state NegResponse_ID
    StateFlowState=7;
  state VersionSendComplete
    ContinueStateProcessing = 0;
    StateFlowState=10;
  note: ?
  state WaitForSWVersionRequest
    StateFlowState=3;
  state SendPos22Resp_SW_Ver [function]
  state SendPos22Resp_SW_Ver1 [function]
  state SendingSoftwareVersionFirstMsg
    StateFlowState=4;
  state SendingSoftwareVersion2ndMsg
  state SendPos11Resp [function]
  state ExitCal
    ContinueStateProcessing = 0;
    StateFlowState=20;
  state WaitForResetRequest
    StateFlowState=5;
  state ECU_Reset [function]
  state ExitLIN_Testing
    ContinueStateProcessing = 0;
    StateFlowState=32;
  state SendingPosResp_ForResetReq
    StateFlowState=6;
  state SendPos31StopPosResp [function]
  state PerformingECU_Reset
    ECU_Reset
    StateFlowState=7;
  state InitializeLIN_Cntrler
    state WriteMODE  % set to Normal Run mode
      StateFlowState= 29;
      en: LIN_Status = SendSPI_3Byte([uint8(0x10),uint8(0b00000000), uint8(0x80)] );
      en: LIN_Status = SendSPI_3Byte([uint8(0xFF),uint8(0b10000000), uint8(0x00)] );
      en: LIN_Status = SendSPI_3Byte([uint8(0x10),uint8(0b10000000), uint8(0x00)] );
    state WriteLIN1_LCFG1 % set to initialization state, write MBL= 20Bits
      StateFlowState= 29;
      en: LIN_Status = SendSPI_3Byte([uint8(0x30),uint8(0b00000000), uint8(0x01)] );
      en: LIN_Status = SendSPI_3Byte([uint8(0x30),uint8(0b00000000), uint8(0b01111001)] );
      en: LIN_Status = SendSPI_3Byte([uint8(0x30),uint8(0b10000000), uint8(0x00)] )
      %WriteBaudRate set baud rate to 20k
      en: LIN_Status5Byte = SendSPI_5Byte([uint8(0x35),uint8(0b00000010), uint8(0x3), uint8(0x72), uint8(0x00) ] );
      en: LIN_Status5Byte = SendSPI_5Byte([uint8(0x35),uint8(0b10000010), uint8(0x0), uint8(0x0), uint8(0x00) ] );
      ;
    state LIN_Status10Byte = SendSPI(SPI_Command1) [function]
    state LIN_Status = SendSPI_3Byte(SPI_Command1) [function]
    state WritePLLCFG % init for 1.832 Mhz Oscillator in Normal mode
      en: LIN_Status = SendSPI_3Byte([uint8(0x30),uint8(0b00000000), uint8(0x00)] );
      en: LIN_Status = SendSPI_3Byte( [uint8(0x01),uint8(0b00000000), uint8(0x4)] )
      en: LIN_Status = SendSPI_3Byte( [uint8(0x01),uint8(0b10000000), uint8(0x0)] );
    state LIN_Status5Byte = SendSPI_5Byte(SPI_Command1) [function]
    state WriteLIN1_LRTC % set RTO to 14 - it is its default value so this step is not necessary
      en: LIN_Status = SendSPI_3Byte([uint8(0x34),uint8(0b00000000), uint8(0xE)]) ;
      en: LIN_Status = SendSPI_3Byte([uint8(0x34),uint8(0b10000000), uint8(0x0)]) ;
    state WriteLIN1_ID
      en: LIN_Status = SendSPI_3Byte([uint8(0x3A),uint8(0b00000000), uint8(0b00101010)] );
      en: LIN_Status = SendSPI_3Byte([uint8(0x3A),uint8(0b10000000), uint8(0x0)] );
    state WriteLIN1_BUF_CTRL % Data Direction = Master TX, 8 Byte TX, Classic Chksum
      en: LIN_Status = SendSPI_3Byte( [uint8(0x3B),uint8(0b00000000), uint8(0b00011111)] );
      en: LIN_Status = SendSPI_3Byte( [uint8(0x3B),uint8(0b10000000), uint8(0x0)] );
    state WriteLIN1_LBD1
      en: LIN_Status10Byte = SendSPI([uint8(0x53),uint8(0b00000111), uint8(0xAA),uint8(0xAA),...
      uint8(0xAA), uint8(0xAA), uint8(0xAA), uint8(0xAA), uint8(0xAA), uint8(0xAA)]) ;
      en: LIN_Status10Byte = SendSPI([uint8(0x53),uint8(0b10000111), uint8(0x0),uint8(0x0),...
      uint8(0x0), uint8(0x0), uint8(0x0), uint8(0x0), uint8(0x0), uint8(0x0)]) ;
    state WriteLIN1_LCFG2 % set to Normal Mode
      %en: LIN_Status = SendSPI_3Byte([uint8(0x30),uint8(0b00000000), uint8(0x00)] );
      %en: LIN_Status = SendSPI_3Byte([uint8(0x30),uint8(0b10000000), uint8(0x00)] );
      en: LIN_Status = SendSPI_3Byte([uint8(0x11),uint8(0b10000000), uint8(0x00)] );
    state WriteLCOM2_ADDR
      en: LIN_Status = SendSPI_3Byte([uint8(0x21),uint8(0b00000000), uint8(0b00000001)] );
    state WriteLIN1_CNTRL
      en: LIN_Status = SendSPI_3Byte( [uint8(0x39),uint8(0b00000000), uint8(0x01)] );
      en: LIN_Status = SendSPI_3Byte( [uint8(0x39),uint8(0b10000000), uint8(0x00)] );
      %en: LIN_Status = SendSPI_3Byte( [uint8(0x21),uint8(0b00000000), uint8(0x01)] );
      %en: LIN_Status = SendSPI_3Byte( [uint8(0x21),uint8(0b10000000), uint8(0x00)] );
      StateFlowState= 31;
    (default) -> WriteMODE  % set to Normal Run mode
    WriteMODE  % set to Normal Run mode -> WriteLIN1_LCFG1 % set to initialization state, write MBL= 20Bits : after(5, msec)
    WriteLIN1_LCFG1 % set to initialization state, write MBL= 20Bits -> WritePLLCFG % init for 1.832 Mhz Oscillator in Normal mode : after(5, msec)
    WritePLLCFG % init for 1.832 Mhz Oscillator in Normal mode -> WriteLIN1_LRTC % set RTO to 14 - it is its default value so this step is not necessary : after(5, msec)
    WriteLIN1_LRTC % set RTO to 14 - it is its default value so this step is not necessary -> WriteLIN1_ID : after(5, msec)
    WriteLIN1_ID -> WriteLIN1_BUF_CTRL % Data Direction = Master TX, 8 Byte TX, Classic Chksum : after(5, msec)
    WriteLIN1_BUF_CTRL % Data Direction = Master TX, 8 Byte TX, Classic Chksum -> WriteLIN1_LBD1 : after(5, msec)
    WriteLIN1_LBD1 -> WriteLIN1_LCFG2 % set to Normal Mode : after(5, msec)
    WriteLIN1_LCFG2 % set to Normal Mode -> WriteLCOM2_ADDR : after(5, msec)
    WriteLCOM2_ADDR -> WriteLIN1_CNTRL : after(5, msec)
    WriteLIN1_CNTRL -> (junction 301)
  state InitializeLIN_Cntrler1
    state ReadRegister
      en: LIN_Status = SendSPI_3Byte([uint8(ServiceByte2),uint8(0b10000000), uint8(0x00)] );
      StateFlowState= 31;
    state LIN_Status = SendSPI_3Byte(SPI_Command1) [function]
    (default) -> ReadRegister
    ReadRegister -> (junction 362)
  PerformingECU_Reset -> Idle : after(1,sec)
  (default) -> Idle
  VersionSendComplete -> Idle
  NegResponse_ID -> Idle : after(500, msec)
  WaitForSWVersionRequest -> Idle [order 2] : after(5, sec)
  ExitLIN_Testing -> Idle
  ExitCal -> Idle : after(20, msec)
  Idle -> ParseMessage : [NewMsgRXed==1]
  ParseMessage -> CalibrateSwitchPack [order 5] : [ (ServiceID == 0x31) && (ServiceByte0==0x01) && (ServiceByte1==0xA1)&& (ServiceByte2==0x02) ]
  ParseMessage -> Diagnostic_ID_req_Verified [order 1] : [ (ServiceID == 0x2E) && (ServiceByte0==0x01) && (ServiceByte1==0x01) ]
  ParseMessage -> InitializeLIN_Cntrler [order 3] : [ (ServiceID == 0x22) && (ServiceByte0==0x01) && (ServiceByte1==0x01) ]
  ParseMessage -> InitializeLIN_Cntrler1 [order 2] : [ (ServiceID == 0x22) && (ServiceByte0==0x01) && (ServiceByte1==0x02)   ]
  ParseMessage -> SW_VersionRequest [order 4] : [ (ServiceID == 0x22) && (ServiceByte0==0x01) && (ServiceByte1==0x00) ]{SendPos22Resp_SW_Ver}
  Diagnostic_ID_req_Verified -> NegResponse_ID [order 2] : [ (ServiceByte2~=0x17) ]{SendNeg2EResponse}
  Diagnostic_ID_req_Verified -> PositiveRespone [order 1] : [ServiceByte2==0x17]{SendPos2EResponse}
  SW_VersionRequest -> VersionSendComplete : {SendPos22Resp_SW_Ver1}
  CalibrateSwitchPack -> ExitCal : [ (ServiceID == 0x31) && (ServiceByte0==0x03) && (ServiceByte1==0xA1) && (ServiceByte2==0x02) ]{SendPos31StopPosResp}
  PositiveRespone -> WaitForSWVersionRequest : after(20, msec)
  WaitForSWVersionRequest -> SendingSoftwareVersionFirstMsg [order 1] : [ (ServiceID == 0x22) && (ServiceByte0==0x01) && (ServiceByte1==0x00) ]{SendPos22Resp_SW_Ver}
  SendingSoftwareVersionFirstMsg -> SendingSoftwareVersion2ndMsg : {SendPos22Resp_SW_Ver1}
  SendingSoftwareVersion2ndMsg -> WaitForResetRequest : after(20, msec)
  WaitForResetRequest -> SendingPosResp_ForResetReq : [ (ServiceID == 0x11) && (ServiceByte0==0x2)]{SendPos11Resp}
  InitializeLIN_Cntrler1 -> ExitLIN_Testing : [StateFlowState==31]
  InitializeLIN_Cntrler -> ExitLIN_Testing : [StateFlowState==31]
  SendingPosResp_ForResetReq -> PerformingECU_Reset : after(500, msec)
  data: SPI_Command1 function_input uint8 size=[1 10]; LIN_Status10Byte function_output uint8 size=[1 10]; SPI_Command1 function_input uint8 size=[1 3]; LIN_Status function_output uint8 size=[1 3]; SPI_Command1 function_input uint8 size=[1 5]; LIN_Status5Byte function_output uint8 size=[1 5]; LIN_Status11Byte1 local uint8 size=[1 11]; SPI_Command1 function_input uint8 size=[1 3]; LIN_Status function_output uint8 size=[1 3]; LIN_Status11Byte1 local uint8 size=[1 11]; ServiceID input; ServiceByte0 input; ServiceByte1 input; ServiceByte2 input uint8 size=1; StateFlowState output uint16; ContinueStateProcessing output uint16; ServiceByte3 input uint8; NewMsgRXed input boolean; LIN_Status output uint8 size=[1 3]; LIN_Status5Byte local uint8 size=[1 5]; LIN_Status10Byte local
